simulink model "S_Function_StateSpaceControllerNominal"  (R2020b)
settings: Solver=VariableStepAuto  StartTime=0.0  StopTime=10.0  RelTol=1e-3
settings Model: Creator=Musta  LastModifiedBy=Musta

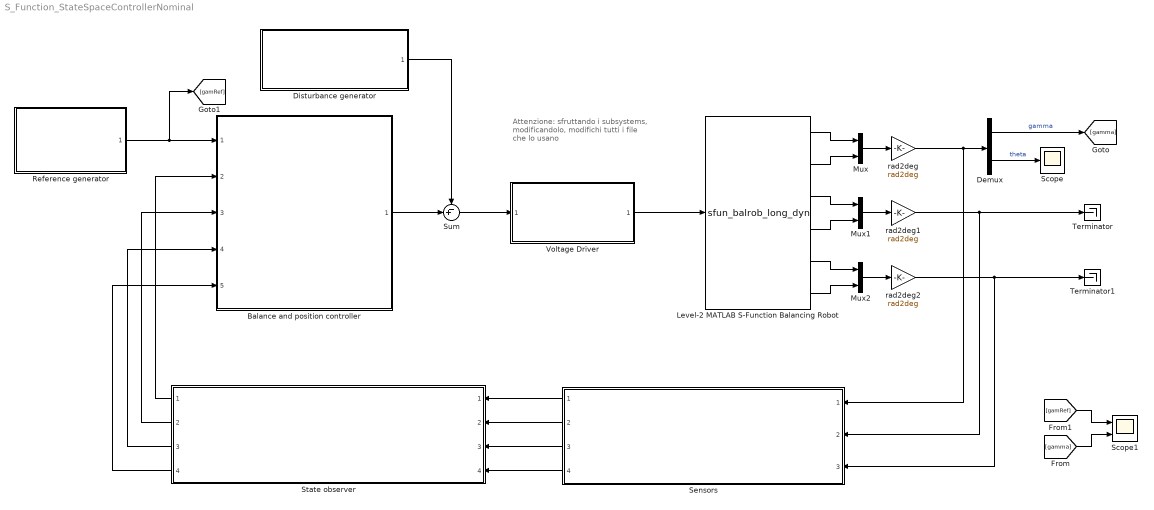
== system S_Function_StateSpaceControllerNominal ==
  note: Attenzione: sfruttando i subsystems, modificandolo, modifichi tutti i file che lo usano
  Balance and position controller : Subsystem  ReferencedSubsystem=StateSpaceControllerNominal_SubSystem
  Demux : Demux  Outputs=2
  Disturbance generator : Subsystem  ReferencedSubsystem=DisturbanceGenerator_SubSystem
  Level-2 MATLAB S-Function Balancing Robot : M-S-Function  FunctionName=sfun_balrob_long_dyn  Parameters=x0 body mot gbox wheel
  Mux : Mux  Inputs=2
  Mux1 : Mux  Inputs=2
  Mux2 : Mux  Inputs=2
  Reference generator : Subsystem  ReferencedSubsystem=GeneratorGam_ref_SubSystem
  Scope : Scope
  Scope1 : Scope  NumInputPorts=2
  Sensors : Subsystem  ReferencedSubsystem=Sensors_SubSystem
      settings: PortSchema="{\"entries\":[{\"content\":{\"sides\":[{\"content\":{\"connectorIds\":[\"Out1\",\"Out2\",\"Out3\",\"Out4\"]},\"type\":\"ConnectorPlacement.EquallySpacedRectSide\",\"uuid\":\"51d9aeda-2f58-468a-8445-73d257530b17\"},{\"content\":{\"connectorIds\":[\"In1\",\"In2\",\"In3\"],\"side\":\"RIGHT\"},\"type\":\"ConnectorPlacement.EquallySpacedRectSide\",\"uuid\":\"77571700-4d1b-47e5-9f8b-52ba036b938f\"},{\"content\":{\"connectorIds\":[],\"side\":\"TOP\"},\"type\":\"ConnectorPlacement.EquallySpacedRectSide\",\"uuid\":\"3da4c363-45f4-4830-b4e0-aa9f00660111\"},{\"content\":{\"connectorIds\":[],\"side\":\"HIDDEN\"},\"type\":\"ConnectorPlacement.EquallySpacedRectSide\",\"uuid\":\"a0dec54f-3332-4ba1-b47c-c34ae4f51399\"}]},\"type\":\"ConnectorPlacement.EquallySpacedConnector\",\"uuid\":\"468e00a1-da97-4578-a7a9-89bb9365fd7e\"}],\"packageUris\":[\"http://schema.mathworks.com/mf0/Connector/R2020b\"],\"version\":\"1.0\"}"
  State observer : Subsystem  ReferencedSubsystem=SimpleStateObserver_SubSystem
  Sum : Sum  Inputs=-+|
  Terminator : Terminator
  Terminator1 : Terminator
  Voltage Driver : Subsystem  ReferencedSubsystem=VoltageDriver_SubSystem
  rad2deg : Gain  Gain=rad2deg
  rad2deg1 : Gain  Gain=rad2deg
  rad2deg2 : Gain  Gain=rad2deg
  wires:
  Level-2 MATLAB S-Function Balancing Robot/2 -> Mux/2
  Level-2 MATLAB S-Function Balancing Robot/1 -> Mux/1
  Level-2 MATLAB S-Function Balancing Robot/3 -> Mux1/1
  Level-2 MATLAB S-Function Balancing Robot/4 -> Mux1/2
  Level-2 MATLAB S-Function Balancing Robot/6 -> Mux2/2
  Level-2 MATLAB S-Function Balancing Robot/5 -> Mux2/1
  Mux2/1 -> rad2deg2/1
  Mux1/1 -> rad2deg1/1
  Mux/1 -> rad2deg/1
  State observer/3 -> Balance and position controller/4
  Sensors/1 -> State observer/1
  Sensors/2 -> State observer/2
  Demux/1 -> [gamma]  "gamma"
  State observer/4 -> Balance and position controller/5
  Sensors/4 -> State observer/4
  Sensors/3 -> State observer/3
  Sum/1 -> Voltage Driver/1
  Demux/2 -> Scope/1  "theta"
  State observer/1 -> Balance and position controller/2
  rad2deg/1 -> Sensors/1, Demux/1
  Reference generator/1 -> [gamRef], Balance and position controller/1
  rad2deg2/1 -> Terminator1/1, Sensors/3
  State observer/2 -> Balance and position controller/3
  Voltage Driver/1 -> Level-2 MATLAB S-Function Balancing Robot/1
  rad2deg1/1 -> Sensors/2, Terminator/1
  Disturbance generator/1 -> Sum/1
  Balance and position controller/1 -> Sum/2
  [gamma] -> Scope1/2
  [gamRef] -> Scope1/1
